simulink library "telecom_lib"  (R2016b)
settings: Solver=VariableStepAuto  StartTime=0.0  StopTime=10.0  RelTol=1e-3
undefined symbols (not defined in the file or in its folder): MET, MET_epoch, sim_params, telecom
libraries: MET_lib x1, bus_stubs_fsw x1
settings Model: Creator=taylorreynolds  LastModifiedBy=taylorreynolds

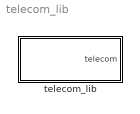
== system telecom_lib ==
  telecom_lib : Subsystem

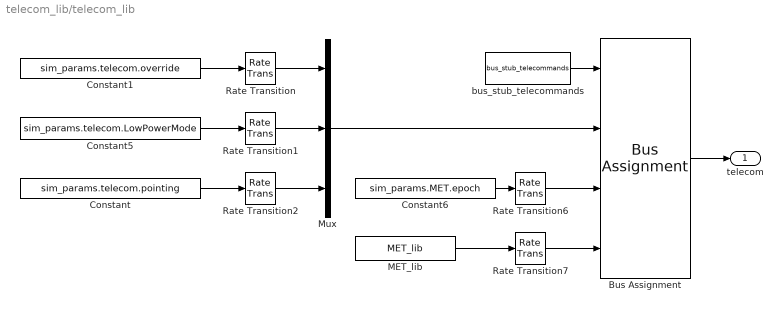
== system telecom_lib/telecom_lib ==
  Bus Assignment : BusAssignment  AssignedSignals=telecom,MET_epoch,MET
  Constant : Constant  Value=sim_params.telecom.pointing  OutDataTypeStr=int8
  Constant1 : Constant  Value=sim_params.telecom.override  OutDataTypeStr=int8
  Constant5 : Constant  Value=sim_params.telecom.LowPowerMode  OutDataTypeStr=int8
  Constant6 : Constant  Value=sim_params.MET.epoch
  MET_lib : MET_lib/MET_lib
  Mux : Mux  Inputs=3
  Rate Transition : RateTransition  X0=sim_params.telecom.ic.override  OutPortSampleTime=sim_params.telecom.sample_time_s
  Rate Transition1 : RateTransition  X0=sim_params.telecom.ic.LowPowerMode  OutPortSampleTime=sim_params.telecom.sample_time_s
  Rate Transition2 : RateTransition  X0=sim_params.telecom.ic.pointing  OutPortSampleTime=sim_params.telecom.sample_time_s
  Rate Transition6 : RateTransition  X0=sim_params.telecom.ic.MET_epoch  OutPortSampleTime=sim_params.telecom.sample_time_s
  Rate Transition7 : RateTransition  OutPortSampleTime=sim_params.telecom.sample_time_s
  bus_stub_telecommands : bus_stubs_fsw/bus_stub_telecommands
  telecom : Outport
  wires:
  Constant1/1 -> Rate Transition/1
  Bus Assignment/1 -> telecom/1
  bus_stub_telecommands/1 -> Bus Assignment/1
  Mux/1 -> Bus Assignment/2
  Rate Transition/1 -> Mux/1
  Constant5/1 -> Rate Transition1/1
  Rate Transition1/1 -> Mux/2
  Rate Transition2/1 -> Mux/3
  Constant/1 -> Rate Transition2/1
  Rate Transition6/1 -> Bus Assignment/3
  Rate Transition7/1 -> Bus Assignment/4
  MET_lib/1 -> Rate Transition7/1
  Constant6/1 -> Rate Transition6/1
